simulink model "B5G_SIM_PDR_ASH_V0"  (R2021a)
settings: Solver=ode4  StartTime=0.0  StopTime=dm.duration  FixedStep=dm.dt  RelTol=1e-3
InitFcn:
  | %b5g_init_param_sdr_v1;
StopFcn:
  | %b5g_post_param_sdr_v1;
  | 
  | %if mdl.OpenAfterSim.sdi
  | %   Simulink.sdi.view;
  | %end
  | 
  | %if mdl.OpenAfterSim.Scope
  | %   open_system(strcat(gcs,'/RateRwTorque'));
  | %end
model workspace (MAT data in the model file):
  RWModelType = 0
values from neighbouring files (symbols this model uses):
  dm = set_dm(dm)    [INIT_B5G_SIM_PDR_ASH.m]
  mdl = set_model_control()    [INIT_B5G_SIM_PDR_ASH.m]    (also in init_b5g_sim_pdr.m = set_model_control('B5G_SIM_PDR_V1'))
  rads2rpm = 60/(2*pi)    (= 9.54929658551)    [INIT_B5G_SIM_PDR_ASH.m]    (also in init_b5g_sim_pdr.m)
undefined symbols (not defined in the file or in its folder): Eclipse, fsw, MagSc, PVeci, Qi2b, RateSc, SunSc
libraries: vrlib x2, aerolibtransform2 x1
(part 2 of 2)

== matlab function B5G_SIM_PDR_ASH_V0/RW_CTRL_FUN/ComputeSaturate ==
  data: T input; Tc output; fsw parameter
function Tc = TorqueSaturation(T, fsw)
T0   = fsw.rw.func.maxTorque;
Trw  = abs(T');
maxT = max(Trw);
if maxT > T0
    Tc = (T0/maxT).*T;
else
    Tc = T;
end
